simulink model "course_2015a"  (R2015a)
settings: Solver=ode3  SolverMode=SingleTasking  StartTime=0.0  StopTime=300  FixedStep=1  RelTol=1e-3
libraries: slctrlblks x1
settings Model: CovMetricSettings=dwe  CovHtmlReporting=off  covSaveCumulativeToWorkspaceVar=off  CovSaveSingleToWorkspaceVar=off  CovExternalEMLEnable=on  Creator=SoloPC  LastModifiedBy=SoloPC
settings DataIOCC: LimitDataPoints=off  SaveFormat=Dataset  ReturnWorkspaceOutputs=on
settings DebuggingCC: SignalRangeChecking=warning  UnconnectedInputMsg=none  UnconnectedOutputMsg=none  UnconnectedLineMsg=none  SFUnexpectedBacktrackingDiag=error  SFNoUnconditionalDefaultTransitionDiag=error
settings HardwareCC: ProdBitPerPointer=64  ProdLargestAtomicFloat=Float  ProdIntDivRoundTo=Zero  ProdEndianess=LittleEndian  ProdHWDeviceType=Specified
settings ModelReferenceCC: PropagateSignalLabelsOutOfModel=on
settings SFSimCC: SimUseLocalCustomCode=on
settings RTWCC: RTWUseLocalCustomCode=on
settings GRTTargetCC: TargetLangStandard=C99 (ISO)

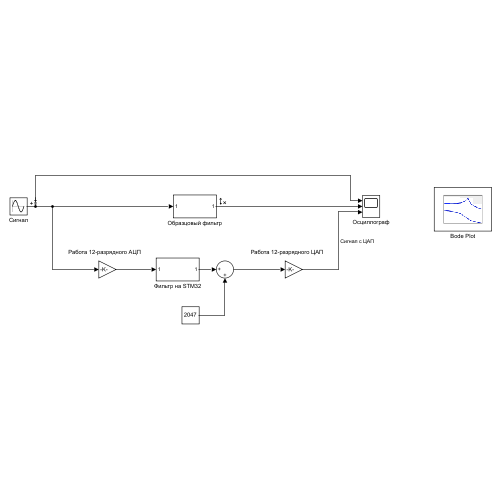
[thumbnail: Simulink's stored preview of the top-level diagram]
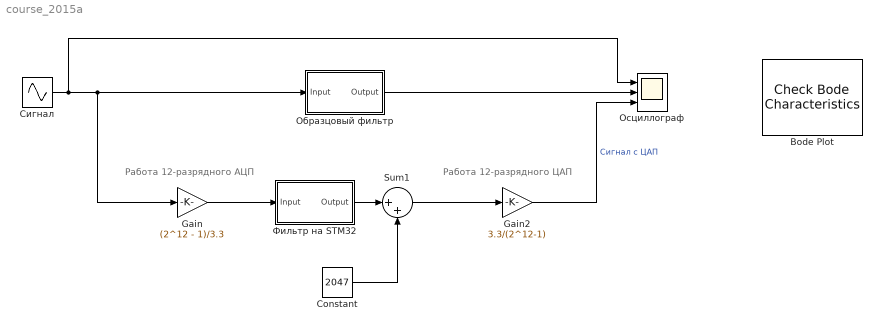
== system course_2015a ==
  note: Работа 12-разрядного АЦП
  note: Работа 12-разрядного ЦАП
  Bode Plot : slctrlblks/Model Verification/Check Bode  Characteristics  InstantiateOnLoad=on  SaveOperatingPoints=off  LinearizationIOs={'/Сигнал', 1, 'in', 'off', '';'/Образцовый фильтр', 1, 'out', 'on', ''}  LinearizeAt=SnapshotTimes  SnapshotTimes=[0]  TriggerType=rising  SampleTime=auto  RateConversionMethod=zoh  PreWarpFreq=10  UseExactDelayModel=off  UseFullBlockNameLabels=off  UseBusSignalLabels=off  enabled=on  stopWhenAssertionFail=off  export=off  ViewDlgPos=[681 157 510 390]  OpenViewOnLoad=off  LaunchViewOnOpen=off  FrequencyUnits=rad/s  MagnitudeUnits=dB  PhaseUnits=deg  TimeUnits=seconds  EnableUpperBound=off  UpperBoundFrequencies=[]  UpperBoundMagnitudes=[]  EnableLowerBound=off  LowerBoundFrequencies=[]  LowerBoundMagnitudes=[]
  Constant : Constant  Value=2047  OutDataTypeStr=double
  Gain : Gain  Gain=(2^12 - 1)/3.3
  Gain2 : Gain  Gain=3.3/(2^12-1)
  Sum1 : Sum  Inputs=|++
  Образцовый фильтр : Subsystem  Tag=FilterWizardSubSystem
      settings: ErrorFcn=dspFilterRealizedInBasicElemsAlgLoopErrFcnCallback
  Осциллограф : Scope  NumInputPorts=3
      settings: TimeRange=auto  ShowLegends=on  MaxDataPoints=5000  SaveToWorkspace=off  SaveName=ScopeData  YMin=-0.25~-1.25766~0.39194  YMax=2.25~1.22956~2.87916  SampleTime=-1
  Сигнал : Sin  Bias=1  Frequency=2 * pi * (500 / 16000)  SampleTime=0
  Фильтр на STM32 : Subsystem  Tag=FilterWizardSubSystem
      settings: ErrorFcn=dspFilterRealizedInBasicElemsAlgLoopErrFcnCallback
  wires:
  Образцовый фильтр/1(Output) -> Осциллограф/2
  Сигнал/1 -> Осциллограф/1, Gain/1, Образцовый фильтр/1(Input)
  Gain/1 -> Фильтр на STM32/1(Input)
  Constant/1 -> Sum1/2
  Gain2/1 -> Осциллограф/3  "Сигнал с ЦАП"
  Фильтр на STM32/1(Output) -> Sum1/1
  Sum1/1 -> Gain2/1

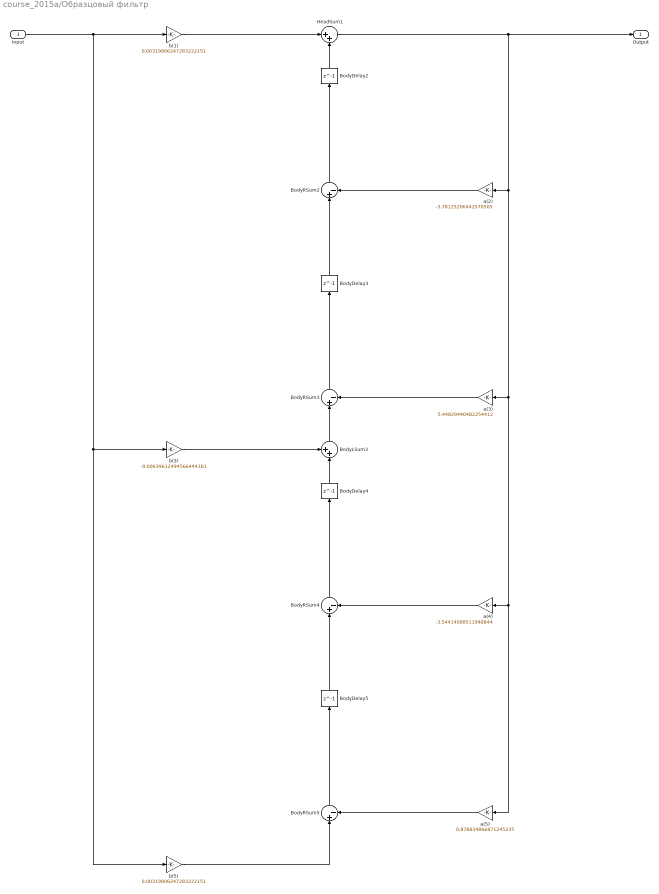
== system course_2015a/Образцовый фильтр ==
  Input : Inport
  BodyDelay{2..5} (4 alike) : Delay  DelayLength=1  InitialCondition=0
  BodyLSum3 : Sum  Inputs=++|  RndMeth=Nearest  SaturateOnIntegerOverflow=on  OutDataTypeStr=Inherit: Same as first input
  BodyRSum{2..5} (4 alike) : Sum  Inputs=|+-  RndMeth=Nearest  SaturateOnIntegerOverflow=on  OutDataTypeStr=Inherit: Same as first input
  HeadSum1 : Sum  Inputs=|++  RndMeth=Nearest  SaturateOnIntegerOverflow=on  OutDataTypeStr=Inherit: Same as first input
  a(2) : Gain  Gain=-3.78125206442570505  ParamDataTypeStr=double  RndMeth=Nearest  SaturateOnIntegerOverflow=on  OutDataTypeStr=Inherit: Same as input
  a(3) : Gain  Gain=5.44829440482254412  ParamDataTypeStr=double  RndMeth=Nearest  SaturateOnIntegerOverflow=on  OutDataTypeStr=Inherit: Same as input
  a(4) : Gain  Gain=-3.54414088511948844  ParamDataTypeStr=double  RndMeth=Nearest  SaturateOnIntegerOverflow=on  OutDataTypeStr=Inherit: Same as input
  a(5) : Gain  Gain=0.878834866871245235  ParamDataTypeStr=double  RndMeth=Nearest  SaturateOnIntegerOverflow=on  OutDataTypeStr=Inherit: Same as input
  b(1) : Gain  Gain=0.00319806247283222151  ParamDataTypeStr=double  RndMeth=Nearest  SaturateOnIntegerOverflow=on  OutDataTypeStr=Inherit: Same as input
  b(3) : Gain  Gain=-0.00639612494566444301  ParamDataTypeStr=double  RndMeth=Nearest  SaturateOnIntegerOverflow=on  OutDataTypeStr=Inherit: Same as input
  b(5) : Gain  Gain=0.00319806247283222151  ParamDataTypeStr=double  RndMeth=Nearest  SaturateOnIntegerOverflow=on  OutDataTypeStr=Inherit: Same as input
  Output : Outport
  wires:
  Input/1 -> b(3)/1, b(5)/1, b(1)/1
  b(1)/1 -> HeadSum1/1
  HeadSum1/1 -> a(4)/1, a(5)/1, a(3)/1, a(2)/1, Output/1
  BodyRSum2/1 -> BodyDelay2/1
  a(2)/1 -> BodyRSum2/2
  BodyDelay2/1 -> HeadSum1/2
  b(3)/1 -> BodyLSum3/1
  BodyLSum3/1 -> BodyRSum3/1
  BodyRSum3/1 -> BodyDelay3/1
  a(3)/1 -> BodyRSum3/2
  BodyDelay3/1 -> BodyRSum2/1
  BodyRSum4/1 -> BodyDelay4/1
  a(4)/1 -> BodyRSum4/2
  BodyDelay4/1 -> BodyLSum3/2
  b(5)/1 -> BodyRSum5/1
  BodyRSum5/1 -> BodyDelay5/1
  a(5)/1 -> BodyRSum5/2
  BodyDelay5/1 -> BodyRSum4/1

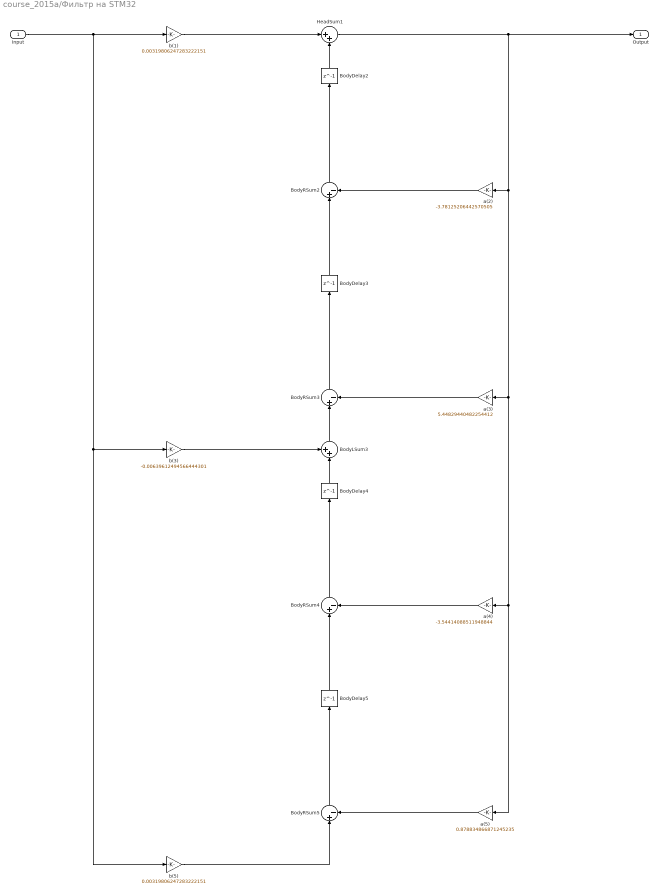
== system course_2015a/Фильтр на STM32 ==
  Input : Inport
  BodyDelay{2..5} (4 alike) : Delay  DelayLength=1  InitialCondition=0
  BodyLSum3 : Sum  Inputs=++|  RndMeth=Nearest  SaturateOnIntegerOverflow=on  OutDataTypeStr=Inherit: Same as first input
  BodyRSum{2..5} (4 alike) : Sum  Inputs=|+-  RndMeth=Nearest  SaturateOnIntegerOverflow=on  OutDataTypeStr=Inherit: Same as first input
  HeadSum1 : Sum  Inputs=|++  RndMeth=Nearest  SaturateOnIntegerOverflow=on  OutDataTypeStr=Inherit: Same as first input
  a(2) : Gain  Gain=-3.78125206442570505  ParamDataTypeStr=double  RndMeth=Nearest  SaturateOnIntegerOverflow=on  OutDataTypeStr=Inherit: Same as input
  a(3) : Gain  Gain=5.44829440482254412  ParamDataTypeStr=double  RndMeth=Nearest  SaturateOnIntegerOverflow=on  OutDataTypeStr=Inherit: Same as input
  a(4) : Gain  Gain=-3.54414088511948844  ParamDataTypeStr=double  RndMeth=Nearest  SaturateOnIntegerOverflow=on  OutDataTypeStr=Inherit: Same as input
  a(5) : Gain  Gain=0.878834866871245235  ParamDataTypeStr=double  RndMeth=Nearest  SaturateOnIntegerOverflow=on  OutDataTypeStr=Inherit: Same as input
  b(1) : Gain  Gain=0.00319806247283222151  ParamDataTypeStr=double  RndMeth=Nearest  SaturateOnIntegerOverflow=on  OutDataTypeStr=Inherit: Same as input
  b(3) : Gain  Gain=-0.00639612494566444301  ParamDataTypeStr=double  RndMeth=Nearest  SaturateOnIntegerOverflow=on  OutDataTypeStr=Inherit: Same as input
  b(5) : Gain  Gain=0.00319806247283222151  ParamDataTypeStr=double  RndMeth=Nearest  SaturateOnIntegerOverflow=on  OutDataTypeStr=Inherit: Same as input
  Output : Outport
  wires:
  Input/1 -> b(3)/1, b(5)/1, b(1)/1
  b(1)/1 -> HeadSum1/1
  HeadSum1/1 -> a(4)/1, a(5)/1, a(3)/1, a(2)/1, Output/1
  BodyRSum2/1 -> BodyDelay2/1
  a(2)/1 -> BodyRSum2/2
  BodyDelay2/1 -> HeadSum1/2
  b(3)/1 -> BodyLSum3/1
  BodyLSum3/1 -> BodyRSum3/1
  BodyRSum3/1 -> BodyDelay3/1
  a(3)/1 -> BodyRSum3/2
  BodyDelay3/1 -> BodyRSum2/1
  BodyRSum4/1 -> BodyDelay4/1
  a(4)/1 -> BodyRSum4/2
  BodyDelay4/1 -> BodyLSum3/2
  b(5)/1 -> BodyRSum5/1
  BodyRSum5/1 -> BodyDelay5/1
  a(5)/1 -> BodyRSum5/2
  BodyDelay5/1 -> BodyRSum4/1
